simulink model "PID_sample"  (R2021a)
settings: Solver=FixedStepAuto  StartTime=0.0  StopTime=50  FixedStep=0.001  RelTol=1e-3
libraries: simulink_extras x1
settings Model: Creator=Lenovo  LastModifiedBy=Lenovo

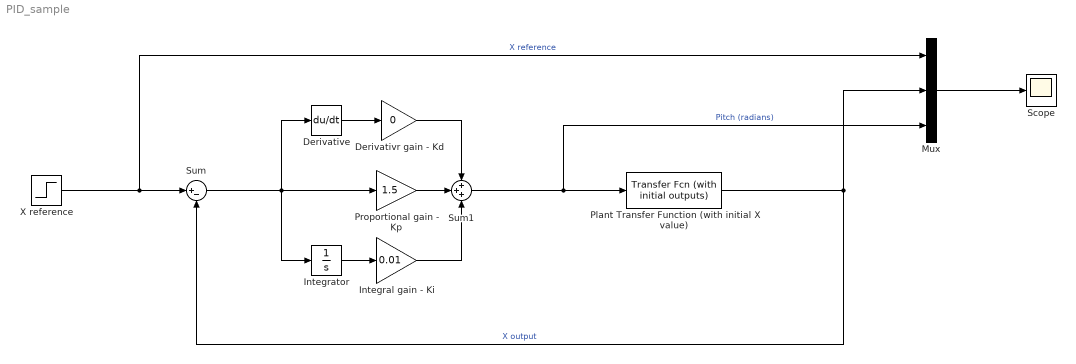
== system PID_sample ==
  Derivative : Derivative
  Derivativr gain - Kd : Gain  Gain=0
  Integral gain - Ki : Gain  Gain=0.01
  Integrator : Integrator
  Mux : Mux  Inputs=3
  Plant Transfer Function (with initial X value) : simulink_extras/Additional Linear/Transfer Fcn (with initial outputs)  N=[13.72]  D=[1 0 0]  Y0=1  U0=0
  Proportional gain - Kp : Gain  Gain=1.5
  "Scope " : Scope
  Sum : Sum  Inputs=|+-
  Sum1 : Sum  Inputs=+++
  X reference : Step  Time=0  After=4  SampleTime=0
  wires:
  Mux/1 -> "Scope "/1
  Proportional gain - Kp/1 -> Sum1/2
  Derivative/1 -> Derivativr gain - Kd/1
  Integrator/1 -> Integral gain - Ki/1
  Derivativr gain - Kd/1 -> Sum1/1
  Integral gain - Ki/1 -> Sum1/3
  Plant Transfer Function (with initial X value)/1 -> Sum/2, Mux/2  "X output"
  Sum1/1 -> Mux/3, Plant Transfer Function (with initial X value)/1  "Pitch (radians)"
  Sum/1 -> Integrator/1, Derivative/1, Proportional gain - Kp/1
  X reference/1 -> Mux/1, Sum/1  "X reference"
